simulink model "logigramme_ds_exo_3"  (R2017b)
settings: Solver=VariableStepAuto  StartTime=0.0  StopTime=8  RelTol=1e-3
libraries: simulink_extras x3
settings Model: Creator=exybore  LastModifiedBy=exybore

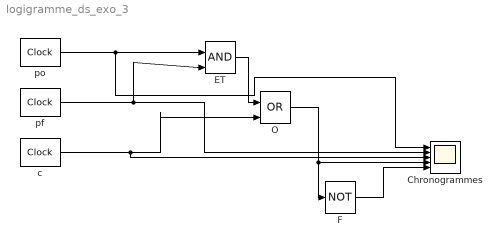
== system logigramme_ds_exo_3 ==
  "Chronogrammes " : Scope  NumInputPorts=5
  ET : Logic  IconShape=distinctive  AllPortsSameDT=off  OutDataTypeStr=boolean
  F : Logic  Operator=NOT  IconShape=distinctive  AllPortsSameDT=off  OutDataTypeStr=boolean
  O : Logic  Operator=OR  IconShape=distinctive  AllPortsSameDT=off  OutDataTypeStr=boolean
  c : simulink_extras/Flip Flops/Clock  period=2
  pf : simulink_extras/Flip Flops/Clock  period=4
  "po " : simulink_extras/Flip Flops/Clock  period=8
  wires:
  O/1 -> F/1, "Chronogrammes "/4
  ET/1 -> O/1
  c/1 -> "Chronogrammes "/3, O/2
  pf/1 -> "Chronogrammes "/2, ET/2
  "po "/1 -> "Chronogrammes "/1, ET/1
  F/1 -> "Chronogrammes "/5
